simulink model "Emergency_Blinking"  (Simulink 8.1)
settings: Solver=ode3  StartTime=0.0  StopTime=10.0  FixedStep=1  RelTol=1e-3
model workspace (MATLAB code in the model file):
  | HAZARD = 1;
  | 
  | LEFT = 2;
  | 
  | RIGHT = 3;
  | 
  | LEFT_AND_RIGHT = 4;
  | 
  | RB_TRUE = 1;
  | 
  | RB_HAZARD = 6;
  | 
  | INDICATORS_OFF = 7;
  | 
  | HAZARD_RB_LEFT = 8;
  | 
  | HAZARD_RB_RIGHT = 9;
settings Model: Creator=CAckermann  LastModifiedBy=cschulze
settings DataIOCC: ExternalInput=testInput  LoadExternalInput=on
settings OptimizationCC: InitFltsAndDblsToZero=on
settings DebuggingCC: SaveWithParameterizedLinksMsg=none  SignalResolutionControl=TryResolveAllWithWarning  MultiTaskDSMMsg=warning  MultiTaskCondExecSysMsg=none  StrictBusMsg=Warning
settings RTWCC: IncludeERTFirstTime=on
settings GRTTargetCC: TargetFcnLib=ansi_tfl_tmw.mat

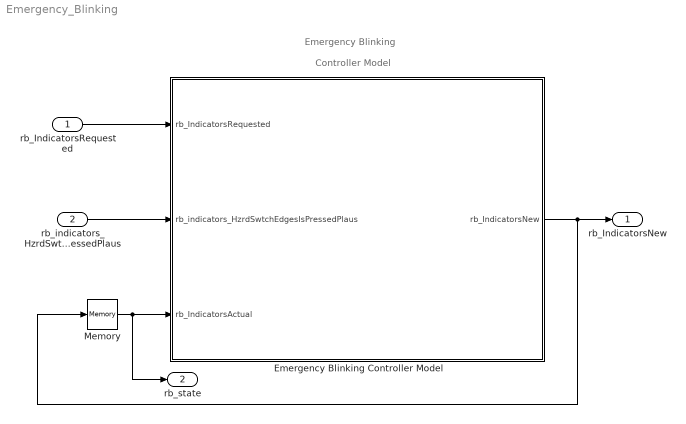
== system Emergency_Blinking ==
  note: Emergency Blinking
  note: Controller Model
  rb_IndicatorsRequested : Inport  OutDataTypeStr=double
  rb_indicators_HzrdSwtchEdgesIsPressedPlaus : Inport  Port=2  OutDataTypeStr=double
  Emergency Blinking Controller Model : Subsystem
  Memory : Memory  X0=7  InheritSampleTime=on
  rb_IndicatorsNew : Outport
  rb_state : Outport  Port=2
  wires:
  rb_IndicatorsRequested/1 -> Emergency Blinking Controller Model/1(rb_IndicatorsRequested)
  rb_indicators_HzrdSwtchEdgesIsPressedPlaus/1 -> Emergency Blinking Controller Model/2(rb_indicators_HzrdSwtchEdgesIsPressedPlaus)
  Emergency Blinking Controller Model/1(rb_IndicatorsNew) -> rb_IndicatorsNew/1, Memory/1
  Memory/1 -> Emergency Blinking Controller Model/3(rb_IndicatorsActual), rb_state/1

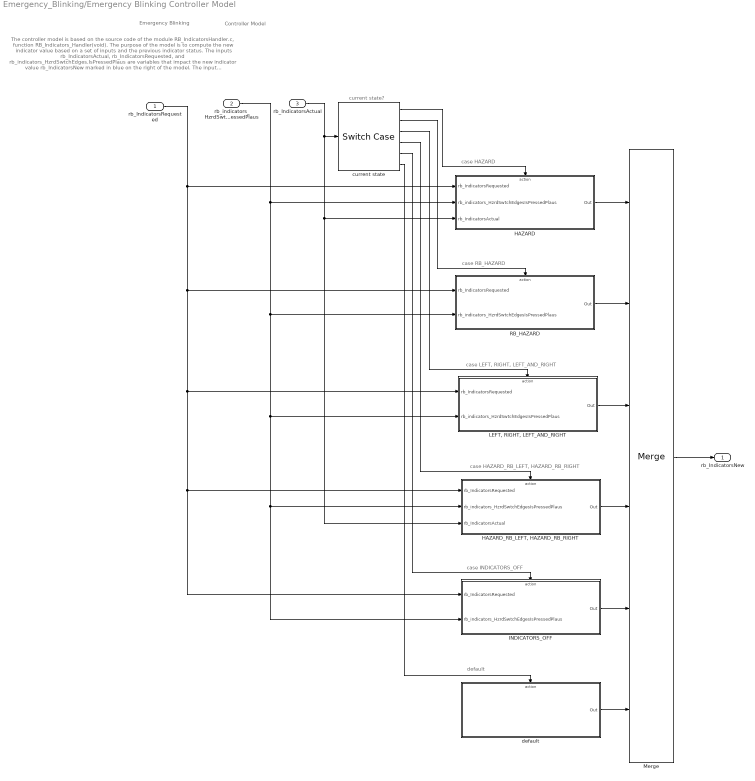
== system Emergency_Blinking/Emergency Blinking Controller Model ==
  note: case HAZARD
  note: case RB_HAZARD
  note: case LEFT, RIGHT, LEFT_AND_RIGHT
  note: case HAZARD_RB_LEFT, HAZARD_RB_RIGHT
  note: case INDICATORS_OFF
  note: default
  note: current state?
  note: The controller model is based on the source code of the module RB_IndicatorsHandler.c, function RB_Indicators_Handler(void).
      | The purpose of the model is to compute the new indicator value based on a set of inputs and the previous indicator status.
      | The inputs rb_IndicatorsActual, rb_IndicatorsRequested, and rb_indicators_HzrdSwtchEdges.IsPressedPlaus are variables that impact the new indicator
      | value rb_IndicatorsNew marked in blue on the right of the model. The input rb_IndicatorsActual is the indicator status of the previous
      | time step whereas rb_IndicatorsRequested and rb_indicators_HzrdSwtchEdges.IsPressedPlaus are values received via CAN.
  note: Emergency Blinking
  note: Controller Model
  rb_IndicatorsRequested : Inport  OutDataTypeStr=double
  rb_indicators_HzrdSwtchEdgesIsPressedPlaus : Inport  Port=2  OutDataTypeStr=double
  rb_IndicatorsActual : Inport  Port=3  OutDataTypeStr=double
  HAZARD : Subsystem  TreatAsAtomicUnit=on
  "HAZARD_RB_LEFT, HAZARD_RB_RIGHT" : Subsystem  TreatAsAtomicUnit=on
  INDICATORS_OFF : Subsystem  TreatAsAtomicUnit=on
  "LEFT, RIGHT, LEFT_AND_RIGHT" : Subsystem  TreatAsAtomicUnit=on
  Merge : Merge  Inputs=6
  RB_HAZARD : Subsystem  TreatAsAtomicUnit=on
  current state : SwitchCase  CaseConditions={HAZARD,RB_HAZARD,[LEFT,RIGHT,LEFT_AND_RIGHT],[HAZARD_RB_LEFT,HAZARD_RB_RIGHT],INDICATORS_OFF}
  default : Subsystem  TreatAsAtomicUnit=on
  rb_IndicatorsNew : Outport
  wires:
  current state/1 -> HAZARD/Action
  rb_IndicatorsActual/1 -> current state/1, HAZARD/3(rb_IndicatorsActual), "HAZARD_RB_LEFT, HAZARD_RB_RIGHT"/3(rb_IndicatorsActual)
  rb_indicators_HzrdSwtchEdgesIsPressedPlaus/1 -> HAZARD/2(rb_indicators_HzrdSwtchEdgesIsPressedPlaus), RB_HAZARD/2(rb_indicators_HzrdSwtchEdgesIsPressedPlaus), "LEFT, RIGHT, LEFT_AND_RIGHT"/2(rb_indicators_HzrdSwtchEdgesIsPressedPlaus), "HAZARD_RB_LEFT, HAZARD_RB_RIGHT"/2(rb_indicators_HzrdSwtchEdgesIsPressedPlaus), INDICATORS_OFF/2(rb_indicators_HzrdSwtchEdgesIsPressedPlaus)
  rb_IndicatorsRequested/1 -> HAZARD/1(rb_IndicatorsRequested), RB_HAZARD/1(rb_IndicatorsRequested), "LEFT, RIGHT, LEFT_AND_RIGHT"/1(rb_IndicatorsRequested), "HAZARD_RB_LEFT, HAZARD_RB_RIGHT"/1(rb_IndicatorsRequested), INDICATORS_OFF/1(rb_IndicatorsRequested)
  current state/2 -> RB_HAZARD/Action
  current state/3 -> "LEFT, RIGHT, LEFT_AND_RIGHT"/Action
  current state/4 -> "HAZARD_RB_LEFT, HAZARD_RB_RIGHT"/Action
  current state/5 -> INDICATORS_OFF/Action
  Merge/1 -> rb_IndicatorsNew/1
  HAZARD/1(Out) -> Merge/1
  RB_HAZARD/1(Out) -> Merge/2
  "LEFT, RIGHT, LEFT_AND_RIGHT"/1(Out) -> Merge/3
  "HAZARD_RB_LEFT, HAZARD_RB_RIGHT"/1(Out) -> Merge/4
  INDICATORS_OFF/1(Out) -> Merge/5
  current state/6 -> default/Action
  default/1(Out) -> Merge/6

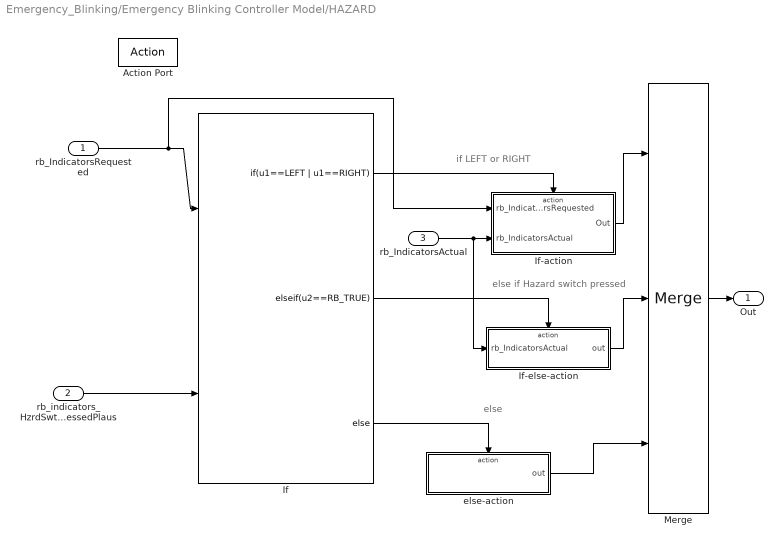
== system Emergency_Blinking/Emergency Blinking Controller Model/HAZARD ==
  note: if LEFT or RIGHT
  note: else if Hazard switch pressed
  note: else
  rb_IndicatorsRequested : Inport  OutDataTypeStr=double
  rb_indicators_HzrdSwtchEdgesIsPressedPlaus : Inport  Port=2  OutDataTypeStr=double
  rb_IndicatorsActual : Inport  Port=3  OutDataTypeStr=double
  Action Port : ActionPort  ActionType=case
  If : If  NumInputs=2  IfExpression=u1==LEFT | u1==RIGHT  ElseIfExpressions=u2==RB_TRUE
  If-action : Subsystem  TreatAsAtomicUnit=on
  If-else-action : Subsystem  TreatAsAtomicUnit=on
  Merge : Merge  Inputs=3
  else-action : Subsystem  TreatAsAtomicUnit=on
  Out : Outport
  wires:
  If/2 -> If-else-action/Action
  If/1 -> If-action/Action
  If/3 -> else-action/Action
  rb_IndicatorsRequested/1 -> If/1, If-action/1(rb_IndicatorsRequested)
  Merge/1 -> Out/1
  rb_IndicatorsActual/1 -> If-action/2(rb_IndicatorsActual), If-else-action/1(rb_IndicatorsActual)
  rb_indicators_HzrdSwtchEdgesIsPressedPlaus/1 -> If/2
  If-action/1(Out) -> Merge/1
  If-else-action/1(out) -> Merge/2
  else-action/1(out) -> Merge/3

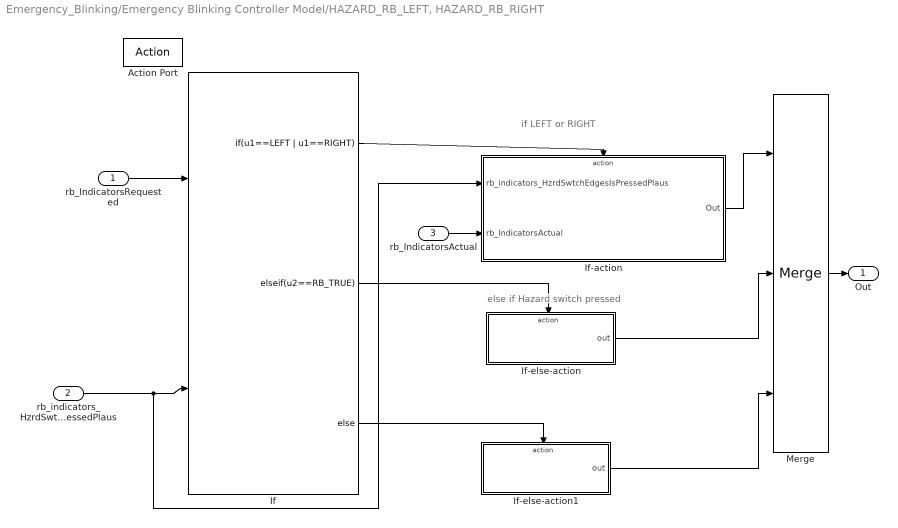
== system Emergency_Blinking/Emergency Blinking Controller Model/HAZARD_RB_LEFT, HAZARD_RB_RIGHT ==
  note: if LEFT or RIGHT
  note: else if Hazard switch pressed
  rb_IndicatorsRequested : Inport  OutDataTypeStr=double
  rb_indicators_HzrdSwtchEdgesIsPressedPlaus : Inport  Port=2  OutDataTypeStr=double
  rb_IndicatorsActual : Inport  Port=3  OutDataTypeStr=double
  Action Port : ActionPort  ActionType=case
  If : If  NumInputs=2  IfExpression=u1==LEFT | u1==RIGHT  ElseIfExpressions=u2==RB_TRUE
  If-action : Subsystem  TreatAsAtomicUnit=on
  If-else-action : Subsystem  TreatAsAtomicUnit=on
  If-else-action1 : Subsystem  TreatAsAtomicUnit=on
  Merge : Merge  Inputs=3
  Out : Outport
  wires:
  If/2 -> If-else-action/Action
  If/1 -> If-action/Action
  rb_IndicatorsRequested/1 -> If/1
  rb_indicators_HzrdSwtchEdgesIsPressedPlaus/1 -> If-action/1(rb_indicators_HzrdSwtchEdgesIsPressedPlaus), If/2
  Merge/1 -> Out/1
  rb_IndicatorsActual/1 -> If-action/2(rb_IndicatorsActual)
  If/3 -> If-else-action1/Action
  If-action/1(Out) -> Merge/1
  If-else-action/1(out) -> Merge/2
  If-else-action1/1(out) -> Merge/3

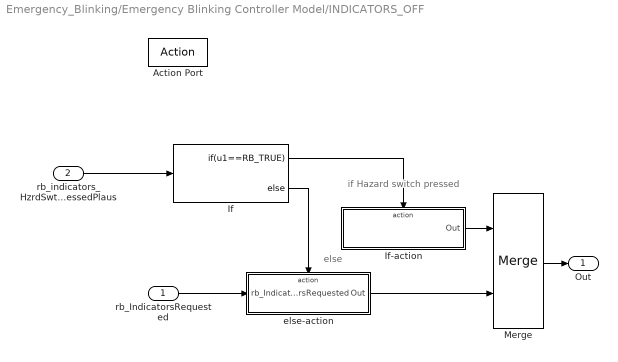
== system Emergency_Blinking/Emergency Blinking Controller Model/INDICATORS_OFF ==
  note: else
  note: if Hazard switch pressed
  rb_IndicatorsRequested : Inport  OutDataTypeStr=double
  rb_indicators_HzrdSwtchEdgesIsPressedPlaus : Inport  Port=2  OutDataTypeStr=double
  Action Port : ActionPort  ActionType=case
  If : If  IfExpression=u1==RB_TRUE
  If-action : Subsystem  TreatAsAtomicUnit=on
  Merge : Merge
  else-action : Subsystem  TreatAsAtomicUnit=on
  Out : Outport
  wires:
  If/1 -> If-action/Action
  If/2 -> else-action/Action
  Merge/1 -> Out/1
  rb_indicators_HzrdSwtchEdgesIsPressedPlaus/1 -> If/1
  rb_IndicatorsRequested/1 -> else-action/1(rb_IndicatorsRequested)
  If-action/1(Out) -> Merge/1
  else-action/1(Out) -> Merge/2

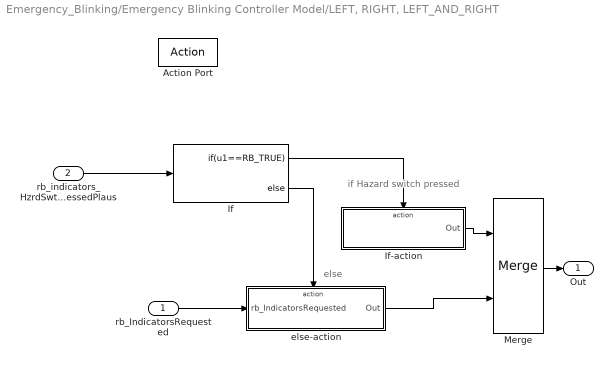
== system Emergency_Blinking/Emergency Blinking Controller Model/LEFT, RIGHT, LEFT_AND_RIGHT ==
  note: else
  note: if Hazard switch pressed
  rb_IndicatorsRequested : Inport  OutDataTypeStr=double
  rb_indicators_HzrdSwtchEdgesIsPressedPlaus : Inport  Port=2  OutDataTypeStr=double
  Action Port : ActionPort  ActionType=case
  If : If  IfExpression=u1==RB_TRUE
  If-action : Subsystem  TreatAsAtomicUnit=on
  Merge : Merge
  else-action : Subsystem  TreatAsAtomicUnit=on
  Out : Outport
  wires:
  If/1 -> If-action/Action
  If/2 -> else-action/Action
  Merge/1 -> Out/1
  rb_indicators_HzrdSwtchEdgesIsPressedPlaus/1 -> If/1
  rb_IndicatorsRequested/1 -> else-action/1(rb_IndicatorsRequested)
  If-action/1(Out) -> Merge/1
  else-action/1(Out) -> Merge/2

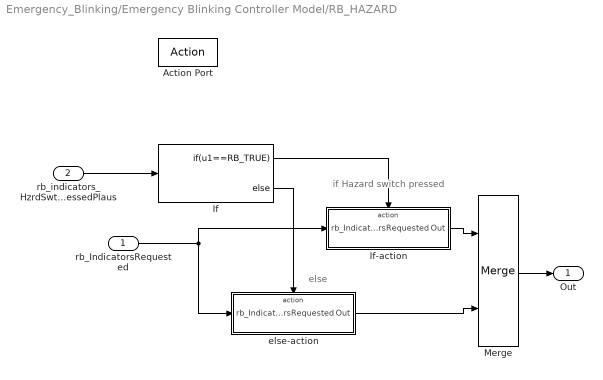
== system Emergency_Blinking/Emergency Blinking Controller Model/RB_HAZARD ==
  note: else
  note: if Hazard switch pressed
  rb_IndicatorsRequested : Inport  OutDataTypeStr=double
  rb_indicators_HzrdSwtchEdgesIsPressedPlaus : Inport  Port=2  OutDataTypeStr=double
  Action Port : ActionPort  ActionType=case
  If : If  IfExpression=u1==RB_TRUE
  If-action : Subsystem  TreatAsAtomicUnit=on
  Merge : Merge
  else-action : Subsystem  TreatAsAtomicUnit=on
  Out : Outport
  wires:
  If/1 -> If-action/Action
  If/2 -> else-action/Action
  Merge/1 -> Out/1
  rb_indicators_HzrdSwtchEdgesIsPressedPlaus/1 -> If/1
  rb_IndicatorsRequested/1 -> If-action/1(rb_IndicatorsRequested), else-action/1(rb_IndicatorsRequested)
  If-action/1(Out) -> Merge/1
  else-action/1(Out) -> Merge/2

== system Emergency_Blinking/Emergency Blinking Controller Model/default ==
  Action Port : ActionPort  ActionType=default
  Default : Constant  Value=INDICATORS_OFF
  Out : Outport
  wires:
  Default/1 -> Out/1

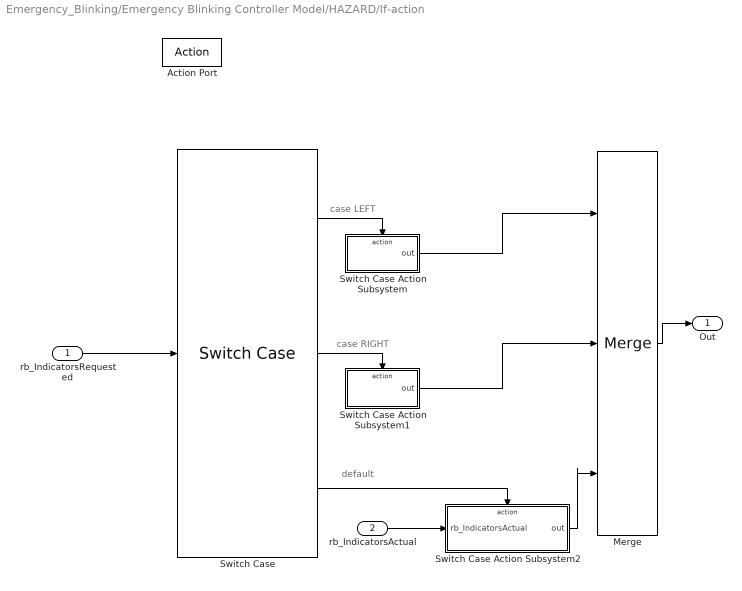
== system Emergency_Blinking/Emergency Blinking Controller Model/HAZARD/If-action ==
  note: case LEFT
  note: case RIGHT
  note: default
  rb_IndicatorsRequested : Inport  OutDataTypeStr=double
  rb_IndicatorsActual : Inport  Port=2  OutDataTypeStr=double
  Action Port : ActionPort  ActionType=then
  Merge : Merge  Inputs=3
  Switch Case : SwitchCase  CaseConditions={LEFT,RIGHT}
  Switch Case Action Subsystem : Subsystem  TreatAsAtomicUnit=on
  Switch Case Action Subsystem1 : Subsystem  TreatAsAtomicUnit=on
  Switch Case Action Subsystem2 : Subsystem  TreatAsAtomicUnit=on
  Out : Outport
  wires:
  Switch Case/1 -> Switch Case Action Subsystem/Action
  Switch Case/2 -> Switch Case Action Subsystem1/Action
  Switch Case/3 -> Switch Case Action Subsystem2/Action
  Merge/1 -> Out/1
  rb_IndicatorsRequested/1 -> Switch Case/1
  rb_IndicatorsActual/1 -> Switch Case Action Subsystem2/1(rb_IndicatorsActual)
  Switch Case Action Subsystem/1(out) -> Merge/1
  Switch Case Action Subsystem1/1(out) -> Merge/2
  Switch Case Action Subsystem2/1(out) -> Merge/3

== system Emergency_Blinking/Emergency Blinking Controller Model/HAZARD/If-else-action ==
  rb_IndicatorsActual : Inport  OutDataTypeStr=double
  Action Port : ActionPort  ActionType=elseif
  out : Outport
  wires:
  rb_IndicatorsActual/1 -> out/1

== system Emergency_Blinking/Emergency Blinking Controller Model/HAZARD/else-action ==
  Action Port : ActionPort  ActionType=else
  Constant3 : Constant  Value=INDICATORS_OFF
  out : Outport
  wires:
  Constant3/1 -> out/1

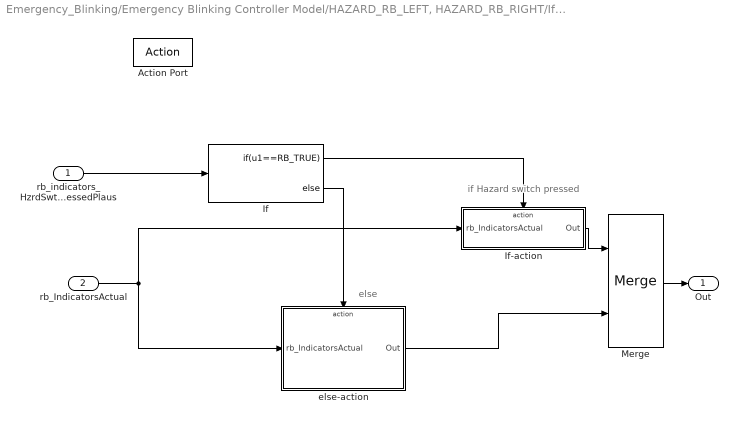
== system Emergency_Blinking/Emergency Blinking Controller Model/HAZARD_RB_LEFT, HAZARD_RB_RIGHT/If-action ==
  note: else
  note: if Hazard switch pressed
  rb_indicators_HzrdSwtchEdgesIsPressedPlaus : Inport  OutDataTypeStr=double
  rb_IndicatorsActual : Inport  Port=2  OutDataTypeStr=double
  Action Port : ActionPort  ActionType=then
  If : If  IfExpression=u1==RB_TRUE
  If-action : Subsystem  TreatAsAtomicUnit=on
  Merge : Merge
  else-action : Subsystem  TreatAsAtomicUnit=on
  Out : Outport
  wires:
  If/1 -> If-action/Action
  If/2 -> else-action/Action
  Merge/1 -> Out/1
  rb_indicators_HzrdSwtchEdgesIsPressedPlaus/1 -> If/1
  rb_IndicatorsActual/1 -> If-action/1(rb_IndicatorsActual), else-action/1(rb_IndicatorsActual)
  If-action/1(Out) -> Merge/1
  else-action/1(Out) -> Merge/2

== system Emergency_Blinking/Emergency Blinking Controller Model/HAZARD_RB_LEFT, HAZARD_RB_RIGHT/If-else-action ==
  Action Port : ActionPort  ActionType=elseif
  Constant2 : Constant  Value=HAZARD
  out : Outport
  wires:
  Constant2/1 -> out/1

== system Emergency_Blinking/Emergency Blinking Controller Model/HAZARD_RB_LEFT, HAZARD_RB_RIGHT/If-else-action1 ==
  Action Port : ActionPort  ActionType=else
  Default : Constant  Value=INDICATORS_OFF
  out : Outport
  wires:
  Default/1 -> out/1

== system Emergency_Blinking/Emergency Blinking Controller Model/INDICATORS_OFF/If-action ==
  Action Port : ActionPort  ActionType=then
  Constant3 : Constant  Value=HAZARD
  Out : Outport
  wires:
  Constant3/1 -> Out/1

== system Emergency_Blinking/Emergency Blinking Controller Model/INDICATORS_OFF/else-action ==
  rb_IndicatorsRequested : Inport  OutDataTypeStr=double
  Action Port : ActionPort  ActionType=else
  Out : Outport
  wires:
  rb_IndicatorsRequested/1 -> Out/1

== system Emergency_Blinking/Emergency Blinking Controller Model/LEFT, RIGHT, LEFT_AND_RIGHT/If-action ==
  Action Port : ActionPort  ActionType=then
  Constant3 : Constant  Value=RB_HAZARD
  Out : Outport
  wires:
  Constant3/1 -> Out/1

== system Emergency_Blinking/Emergency Blinking Controller Model/LEFT, RIGHT, LEFT_AND_RIGHT/else-action ==
  rb_IndicatorsRequested : Inport  OutDataTypeStr=double
  Action Port : ActionPort  ActionType=else
  Out : Outport
  wires:
  rb_IndicatorsRequested/1 -> Out/1

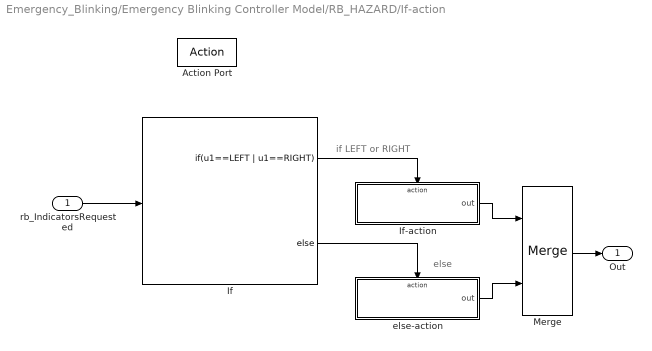
== system Emergency_Blinking/Emergency Blinking Controller Model/RB_HAZARD/If-action ==
  note: if LEFT or RIGHT
  note: else
  rb_IndicatorsRequested : Inport  OutDataTypeStr=double
  Action Port : ActionPort  ActionType=then
  If : If  IfExpression=u1==LEFT | u1==RIGHT
  If-action : Subsystem  TreatAsAtomicUnit=on
  Merge : Merge
  else-action : Subsystem  TreatAsAtomicUnit=on
  Out : Outport
  wires:
  If/1 -> If-action/Action
  If/2 -> else-action/Action
  rb_IndicatorsRequested/1 -> If/1
  Merge/1 -> Out/1
  If-action/1(out) -> Merge/1
  else-action/1(out) -> Merge/2

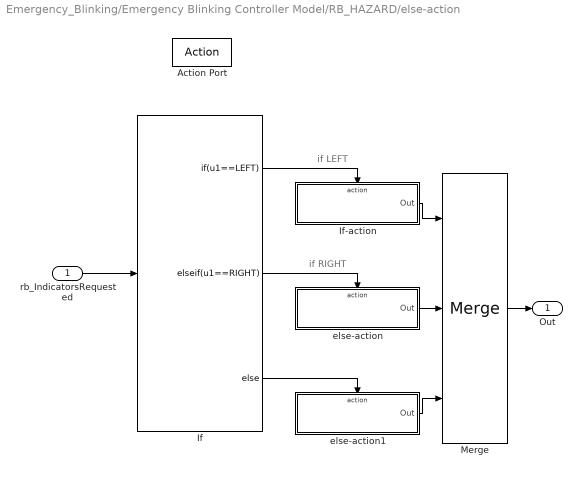
== system Emergency_Blinking/Emergency Blinking Controller Model/RB_HAZARD/else-action ==
  note: if LEFT
  note: if RIGHT
  rb_IndicatorsRequested : Inport  OutDataTypeStr=double
  Action Port : ActionPort  ActionType=else
  If : If  IfExpression=u1==LEFT  ElseIfExpressions=u1==RIGHT
  If-action : Subsystem  TreatAsAtomicUnit=on
  Merge : Merge  Inputs=3
  else-action : Subsystem  TreatAsAtomicUnit=on
  else-action1 : Subsystem  TreatAsAtomicUnit=on
  Out : Outport
  wires:
  rb_IndicatorsRequested/1 -> If/1
  Merge/1 -> Out/1
  If/2 -> else-action/Action
  If/1 -> If-action/Action
  If/3 -> else-action1/Action
  If-action/1(Out) -> Merge/1
  else-action/1(Out) -> Merge/2
  else-action1/1(Out) -> Merge/3

== system Emergency_Blinking/Emergency Blinking Controller Model/HAZARD/If-action/Switch Case Action Subsystem ==
  Action Port : ActionPort  ActionType=case
  Constant111 : Constant  Value=HAZARD_RB_LEFT
  out : Outport
  wires:
  Constant111/1 -> out/1

== system Emergency_Blinking/Emergency Blinking Controller Model/HAZARD/If-action/Switch Case Action Subsystem1 ==
  Action Port : ActionPort  ActionType=case
  Constant3 : Constant  Value=HAZARD_RB_RIGHT
  out : Outport
  wires:
  Constant3/1 -> out/1

== system Emergency_Blinking/Emergency Blinking Controller Model/HAZARD/If-action/Switch Case Action Subsystem2 ==
  rb_IndicatorsActual : Inport  OutDataTypeStr=double
  Action Port : ActionPort  ActionType=default
  out : Outport
  wires:
  rb_IndicatorsActual/1 -> out/1

== system Emergency_Blinking/Emergency Blinking Controller Model/HAZARD_RB_LEFT, HAZARD_RB_RIGHT/If-action/If-action ==
  rb_IndicatorsActual : Inport  OutDataTypeStr=double
  Action Port : ActionPort  ActionType=then
  Out : Outport
  wires:
  rb_IndicatorsActual/1 -> Out/1

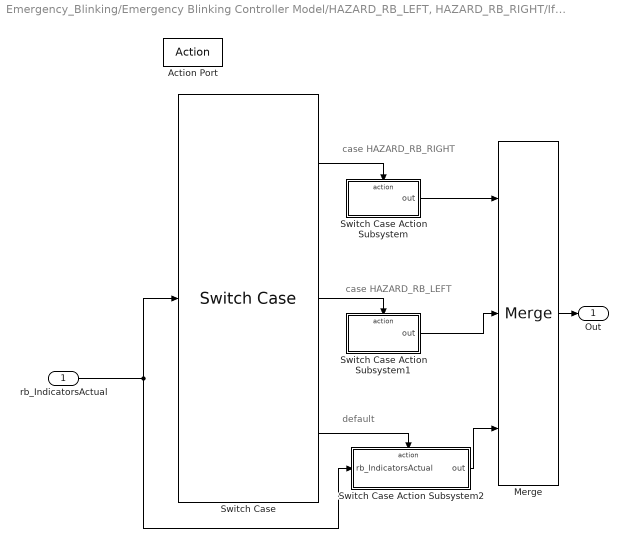
== system Emergency_Blinking/Emergency Blinking Controller Model/HAZARD_RB_LEFT, HAZARD_RB_RIGHT/If-action/else-action ==
  note: case HAZARD_RB_LEFT
  note: case HAZARD_RB_RIGHT
  note: default
  rb_IndicatorsActual : Inport  OutDataTypeStr=double
  Action Port : ActionPort  ActionType=else
  Merge : Merge  Inputs=3
  Switch Case : SwitchCase  CaseConditions={HAZARD_RB_RIGHT,HAZARD_RB_LEFT}
  Switch Case Action Subsystem : Subsystem  TreatAsAtomicUnit=on
  Switch Case Action Subsystem1 : Subsystem  TreatAsAtomicUnit=on
  Switch Case Action Subsystem2 : Subsystem  TreatAsAtomicUnit=on
  Out : Outport
  wires:
  Switch Case/1 -> Switch Case Action Subsystem/Action
  Switch Case/2 -> Switch Case Action Subsystem1/Action
  Switch Case/3 -> Switch Case Action Subsystem2/Action
  Merge/1 -> Out/1
  rb_IndicatorsActual/1 -> Switch Case Action Subsystem2/1(rb_IndicatorsActual), Switch Case/1
  Switch Case Action Subsystem/1(out) -> Merge/1
  Switch Case Action Subsystem1/1(out) -> Merge/2
  Switch Case Action Subsystem2/1(out) -> Merge/3

== system Emergency_Blinking/Emergency Blinking Controller Model/RB_HAZARD/If-action/If-action ==
  Action Port : ActionPort  ActionType=then
  Constant3 : Constant  Value=RB_HAZARD
  out : Outport
  wires:
  Constant3/1 -> out/1

== system Emergency_Blinking/Emergency Blinking Controller Model/RB_HAZARD/If-action/else-action ==
  Action Port : ActionPort  ActionType=else
  Constant3 : Constant  Value=HAZARD
  out : Outport
  wires:
  Constant3/1 -> out/1

== system Emergency_Blinking/Emergency Blinking Controller Model/RB_HAZARD/else-action/If-action ==
  Action Port : ActionPort  ActionType=then
  Constant3 : Constant  Value=LEFT
  Out : Outport
  wires:
  Constant3/1 -> Out/1

== system Emergency_Blinking/Emergency Blinking Controller Model/RB_HAZARD/else-action/else-action ==
  Action Port : ActionPort  ActionType=elseif
  Constant3 : Constant  Value=RIGHT
  Out : Outport
  wires:
  Constant3/1 -> Out/1

== system Emergency_Blinking/Emergency Blinking Controller Model/RB_HAZARD/else-action/else-action1 ==
  Action Port : ActionPort  ActionType=else
  Default : Constant  Value=INDICATORS_OFF
  Out : Outport
  wires:
  Default/1 -> Out/1

== system Emergency_Blinking/Emergency Blinking Controller Model/HAZARD_RB_LEFT, HAZARD_RB_RIGHT/If-action/else-action/Switch Case Action Subsystem ==
  Action Port : ActionPort  ActionType=case
  Constant3 : Constant  Value=RIGHT
  out : Outport
  wires:
  Constant3/1 -> out/1

== system Emergency_Blinking/Emergency Blinking Controller Model/HAZARD_RB_LEFT, HAZARD_RB_RIGHT/If-action/else-action/Switch Case Action Subsystem1 ==
  Action Port : ActionPort  ActionType=case
  Constant3 : Constant  Value=LEFT
  out : Outport
  wires:
  Constant3/1 -> out/1

== system Emergency_Blinking/Emergency Blinking Controller Model/HAZARD_RB_LEFT, HAZARD_RB_RIGHT/If-action/else-action/Switch Case Action Subsystem2 ==
  rb_IndicatorsActual : Inport  OutDataTypeStr=double
  Action Port : ActionPort  ActionType=default
  out : Outport
  wires:
  rb_IndicatorsActual/1 -> out/1
